simulink model "Control_test"  (R2014b)
settings: Solver=FixedStepDiscrete  StartTime=0.0  StopTime=Inf  FixedStep=0.001  RelTol=1e-3
PostLoadFcn:
  | , if any(exist('dsrtsu_mdlpostloadfcn', 'file') == [2, 3, 6]), try dsrtsu_mdlpostloadfcn('Execute', bdroot); catch fprintf('Error in PostLoadFcn (dsrtsu_mdlpostloadfcn) for model "%s":\n %s\n', bdroot, lasterr); end, end,
undefined symbols (not defined in the file or in its folder): dtLocal, slcm
libraries: rtican x163, simulink x14
(part 25 of 34)

== system Control_test/InputProcessing/RadarCanProcessing/Track39 ==
  Bus Creator : BusCreator  Inputs=12
  ESR_Track39 : rtican/RTICAN Receive (RX)   Reserved1=[]  Reserved2=[]  Reserved3=[]  Reserved4=[]  SfcnMessage=[]  Msg_Struct=[]  BoardTypeNo=[]  BoardNo=[]  ChannelNo=[]  Parameters=[]  DialogFcn=[]  UnitName=[]  Revision=[]  UnitValues=[]  DSProperties=struct('RTI',struct('Version',uint32(5),'BlockType',struct('isSLSource',uint8(1),'isSLSink',uint8(1),'isHWSource',uint8(0),'isHWSink',uint8(0),'isSetup',uint8(0),'isInline',uint8(1),'isNonInline',uint8(0),'isInterrupt',uint8(0),'isChannelwise',uint8(0)),'IOBoardType','RTICAN','UnitType','MESSAGE','Identifier','RX','DialogType','MSVC','BlockSet','RTICAN','SlaveProcessor','CAN'))  RTIBlockInterface=struct('OutputPortsWidth',int32([1 1 1 1 1 1 1 1 1 1 1 1]),'OutputPortsActive',[1 1 1 1 1 1 1 1 1 1 1 1],'OutputPortsName',{{'CAN_TX_TRACK_RANGE_RATE_39','CAN_TX_TRACK_MED_RANGE_MODE_39','CAN_TX_TRACK_RANGE_ACCEL_39','CAN_TX_TRACK_WIDTH_39','CAN_TX_TRACK_ROLLING_COUNT_39','CAN_TX_TRACK_BRIDGE_OBJECT_39','CAN_TX_TRACK_RANGE_39','CAN_TX_TRACK_ANGLE_39','CAN_TX_TRACK_STATUS_39','CAN_TX_TRACK_ONCOMING_39','CAN_TX_TRACK_GROUPING_CHANGED_39','CAN_TX_TRACK_LAT_RATE_39'}},'OutputPortsDataType',{{'SS_DOUBLE','SS_DOUBLE','SS_DOUBLE','SS_DOUBLE','SS_DOUBLE','SS_DOUBLE','SS_DOUBLE','SS_DOUBLE','SS_DOUBLE','SS_DOUBLE','SS_DOUBLE','SS_DOUBLE'}},'OutputPortsLabel',{{'CAN_TX_TRACK_RANGE_RATE_39','CAN_TX_TRACK_MED_RANGE_MODE_39','CAN_TX_TRACK_RANGE_ACCEL_39','CAN_TX_TRACK_WIDTH_39','CAN_TX_TRACK_ROLLING_COUNT_39','CAN_TX_TRACK_BRIDGE_OBJECT_39','CAN_TX_TRACK_RANGE_39','CAN_TX_TRACK_ANGLE_39','CAN_TX_TRACK_STATUS_39','CAN_TX_TRACK_ONCOMING_39','CAN_TX_TRACK_GROUPING_CHANGED_39','CAN_TX_TRACK_LAT_RATE_39'}},'OutputPortsLabelMode','ON','InputPortsWidth',int32(0),'InputPortsActive',0,'DialogFcn','rtican_message_interface_gui','BlockDisplay',{{'','center'}},'IconTransparency','on','ParameterTunableNames',{{}},'InitLevel',3,'BlockName',struct('Token',{{'ESR_Track39'}}),'SampleTime',{{0.01}},'TriggerPort',{{'none'}},'EnablePort',{{'none'}})  RTIBlockParameters=struct('BoardTypeNo',{{1,'OFF',[]}},'BoardNo',{{2,'ON',[1 16]}},'ChannelNo',{{2,'ON',[1 2]}},'Parameters',{{struct('DataFileSupport',struct('DataFileSelectedMaster',1,'DataFileSelectedLocal',0,'DataFileName','c:\users\mpc_car\documents\github\mpc-car\controller\dbcfiles\esr_dv3_64tgt.dbc|','DataFileDate',{{{['02-Nov-2012 20:32:52']},{['21-Mar-2013 13:39:53']},{['28-Sep-2011 17:08:52']}}},'SelectedFile',['<no file selected>'],'InterfaceFcn','rtican_dbc_file_parser'),'Options',struct('StatusSelected',0,'TimeSelected',0,'DeltaTimeSelected',0,'BytePortSelected',0,'MessageLengthSelected',0,'TriggerPort',struct('Selected',0,'TriggerType',0),'UserCoding',struct('Selected',0,'InterfaceFile','UserDecodingFile','FcnName','UserDecodeFcn','InportSelected',0,'InportWidth',1,'OutportSelected',0,'OutportWidth',1),'EnablePortSelected',0,'SignalOnPortnameSelected',1,'UseRXService',0),'Message',struct('MsgOnBlocknameSelected',1,'MsgName','ESR_Track39','MsgIdFormat',0,'MsgId',1318,'MsgLength',8,'NumSignals',12,'SampleTime',0.01,'Signal',struct('SgnName',{'CAN_TX_TRACK_RANGE_RATE_39','CAN_TX_TRACK_MED_RANGE_MODE_39','CAN_TX_TRACK_RANGE_ACCEL_39','CAN_TX_TRACK_WIDTH_39','CAN_TX_TRACK_ROLLING_COUNT_39','CAN_TX_TRACK_BRIDGE_OBJECT_39','CAN_TX_TRACK_RANGE_39','CAN_TX_TRACK_ANGLE_39','CAN_TX_TRACK_STATUS_39','CAN_TX_TRACK_ONCOMING_39','CAN_TX_TRACK_GROUPING_CHANGED_39','CAN_TX_TRACK_LAT_RATE_39'},'SgnStartBit',{0,14,16,26,30,31,32,43,53,56,57,58},'SgnLength',{14,2,10,4,1,1,11,10,3,1,1,6},'SgnType',{0,0,0,0,0,0,0,0,0,0,0,0},'ModeValue',{-1,-1,-1,-1,-1,-1,-1,-1,-1,-1,-1,-1},'DataType',{1,0,1,0,0,0,0,1,0,0,0,1},'ByteLayout',{2,2,2,2,2,2,2,2,2,2,2,2},'Factor',{0.01,1,0.05,0.5,1,1,0.1,0.1,1,1,1,0.25},'Offset',{0,0,0,0,0,0,0,0,0,0,0,0},'SgnComment',{{''},{''},{''},{''},{''},{''},{''},{''},{''},{''},{''},{''}},'SgnUnit',{'m/s','','m/s/s','m','','','m','deg','','','',''},'Min',{-81.92,0,-25.6,0,0,0,0,-51.2,0,0,0,-8},'Max',{81.91,3,25.55,7.5,1,0,204.7,51.1,7,0,0,7.75},'SLDataType',{'SS_DOUBLE','SS_DOUBLE','SS_DOUBLE','SS_DOUBLE','SS_DOUBLE','SS_DOUBLE','SS_DOUBLE','SS_DOUBLE','SS_DOUBLE','SS_DOUBLE','SS_DOUBLE','SS_DOUBLE'}),'MsgIdNumFormat',0,'MsgComment',{{''}}),'Version',1.2,'general',struct('isFromLib',0)),'OFF',[]}},'GroupId',{{struct('Group',{{'RTICAN'}},'No',4,'Behavior',{{'NAMECHANGE'}},'BlockType',{{'SINK'}},'NameChangeFlag',0),'OFF',[]}},'SFcnRTICANMessage',{{struct('MsgType','RX','SFcnPortType','Scalar','MsgName','ESR_Track39','MsgIdFormat','STD','MsgId',1318,'MsgLength',8,'NumSignals',12,'SampleTime',0.01,'Signal',struct('SgnName',{'CAN_TX_TRACK_RANGE_RATE_39','CAN_TX_TRACK_MED_RANGE_MODE_39','CAN_TX_TRACK_RANGE_ACCEL_39','CAN_TX_TRACK_WIDTH_39','CAN_TX_TRACK_ROLLING_COUNT_39','CAN_TX_TRACK_BRIDGE_OBJECT_39','CAN_TX_TRACK_RANGE_39','CAN_TX_TRACK_ANGLE_39','CAN_TX_TRACK_STATUS_39','CAN_TX_TRACK_ONCOMING_39','CAN_TX_TRACK_GROUPING_CHANGED_39','CAN_TX_TRACK_LAT_RATE_39'},'SgnStartBit',{0,14,16,26,30,31,32,43,53,56,57,58},'SgnLength',{14,2,10,4,1,1,11,10,3,1,1,6},'SgnType',{'standard','standard','standard','standard','standard','standard','standard','standard','standard','standard','standard','standard'},'ModeValue',{-1,-1,-1,-1,-1,-1,-1,-1,-1,-1,-1,-1},'DataType',{['signed int'],['unsigned int'],['signed int'],['unsigned int'],['unsigned int'],['unsigned int'],['unsigned int'],['signed int'],['unsigned int'],['unsigned int'],['unsigned int'],['signed int']},'ByteLayout',{['motorola back.'],['motorola back.'],['motorola back.'],['motorola back.'],['motorola back.'],['motorola back.'],['motorola back.'],['motorola back.'],['motorola back.'],['motorola back.'],['motorola back.'],['motorola back.']},'Factor',{0.01,1,0.05,0.5,1,1,0.1,0.1,1,1,1,0.25},'Offset',{0,0,0,0,0,0,0,0,0,0,0,0},'SLDataType',{'SS_DOUBLE','SS_DOUBLE','SS_DOUBLE','SS_DOUBLE','SS_DOUBLE','SS_DOUBLE','SS_DOUBLE','SS_DOUBLE','SS_DOUBLE','SS_DOUBLE','SS_DOUBLE','SS_DOUBLE'}),'StatusSelected','no','TimeSelected','no','DeltaTimeSelected','no','BytePortSelected','no','MessageLengthSelected','no','TriggerPort',struct('Selected','no','TriggerType',0),'UserCoding',struct('Selected','no','InterfaceFile','UserDecodingFile','FcnName','UserDecodeFcn','InportSelected','no','InportWidth',1,'OutportSelected','no','OutportWidth',1),'EnablePortSelected','no','UseRXService','no','BoardType','DS1','BoardNo',2,'ControllerNo',2),'OFF',[]}},'TLCFileName',{{'rtican_rx_message','OFF',[]}})  RTISFcnParameters=struct('SFcnRTICANMessage','struct','TLCFileName','char')  RTIBlockParaDefault=struct('BoardTypeNo',4302,'BoardNo',1,'ChannelNo',1,'Parameters',struct('DataFileSupport',struct('DataFileSelectedMaster',0,'DataFileSelectedLocal',0,'DataFileName','','DataFileDate','','SelectedFile',['<no file selected>']),'Options',struct('StatusSelected',1,'TimeSelected',1,'DeltaTimeSelected',1,'BytePortSelected',0,'MessageLengthSelected',0,'TriggerPort',struct('Selected',0,'TriggerType','rising'),'UserCoding',struct('Selected',0,'InterfaceFile','UserDecodingFile','FcnName','UserDecodeFcn','InportSelected',0,'InportWidth',1,'OutportSelected',0,'OutportWidth',1),'EnablePortSelected',0,'SignalOnPortnameSelected',1,'UseRXService',0),'Message',struct('MsgOnBlocknameSelected',0,'MsgName',['RX Message'],'MsgIdFormat',0,'MsgId',100,'MsgLength',8,'NumSignals',1,'SampleTime',-1,'Signal',struct('SgnName',['RX signal'],'SgnStartBit',0,'SgnLength',8,'SgnType',0,'ModeValue',-1,'DataType',0,'SLDataType','SS_DOUBLE','ByteLayout',0,'Factor',1,'Offset',0,'Min',0,'Max',255,'SgnComment',{{}},'SgnUnit',''),'MsgIdNumFormat',0,'MsgComment',{{''}}),'Version',1.2,'general',struct('isFromLib',1)),'GroupId',struct('Group',{{'RTICAN'}},'No',1,'Behavior',{{'NAMECHANGE'}},'BlockType',{{'SINK'}},'NameChangeFlag',0),'SFcnRTICANMessage',struct('MsgType','RX','MsgName',['RX Message'],'MsgIdFormat','STD','MsgId',100,'MsgLength',8,'NumSignals',1,'SampleTime',-1,'Signal',struct('SgnName',['RX signal'],'SgnStartBit',0,'SgnLength',8,'SgnType','standard','ModeValue',-1,'DataType',['unsigned int'],'ByteLayout',['little endian'],'SLDataType','SS_DOUBLE','Factor',1,'Offset',0),'StatusSelected','yes','TimeSelected','yes','DeltaTimeSelected','yes','BytePortSelected','no','MessageLengthSelected','no','EnablePortSelected','no','UserCoding',struct('Selected','no','InterfaceFile','UserDecodingFile','FcnName','UserDecodeFcn','InportSelected','no','InportWidth',1,'OutportSelected','no','OutportWidth',1),'TriggerPort',struct('Selected','no','TriggerType','rising'),'UseRXService','no','BoardType','DS4302','BoardNo',1,'ControllerNo',1,'SFcnPortType','Scalar'),'TLCFileName','rtican_rx_message')
      settings: AttributesFormatString=Group Id: RTICAN4\n
  Out1 : Outport
  wires:
  Bus Creator/1 -> Out1/1  "Track39"
  ESR_Track39/1 -> Bus Creator/1  "CAN_TX_TRACK_RANGE_RATE_39"
  ESR_Track39/2 -> Bus Creator/2  "CAN_TX_TRACK_MED_RANGE_MODE_39"
  ESR_Track39/3 -> Bus Creator/3  "CAN_TX_TRACK_RANGE_ACCEL_39"
  ESR_Track39/4 -> Bus Creator/4  "CAN_TX_TRACK_WIDTH_39"
  ESR_Track39/5 -> Bus Creator/5  "CAN_TX_TRACK_ROLLING_COUNT_39"
  ESR_Track39/6 -> Bus Creator/6  "CAN_TX_TRACK_BRIDGE_OBJECT_39"
  ESR_Track39/7 -> Bus Creator/7  "CAN_TX_TRACK_RANGE_39"
  ESR_Track39/8 -> Bus Creator/8  "CAN_TX_TRACK_ANGLE_39"
  ESR_Track39/9 -> Bus Creator/9  "CAN_TX_TRACK_STATUS_39"
  ESR_Track39/10 -> Bus Creator/10  "CAN_TX_TRACK_ONCOMING_39"
  ESR_Track39/11 -> Bus Creator/11  "CAN_TX_TRACK_GROUPING_CHANGED_39"
  ESR_Track39/12 -> Bus Creator/12  "CAN_TX_TRACK_LAT_RATE_39"

== system Control_test/InputProcessing/RadarCanProcessing/Track40 ==
  Bus Creator : BusCreator  Inputs=12
  ESR_Track40 : rtican/RTICAN Receive (RX)   Reserved1=[]  Reserved2=[]  Reserved3=[]  Reserved4=[]  SfcnMessage=[]  Msg_Struct=[]  BoardTypeNo=[]  BoardNo=[]  ChannelNo=[]  Parameters=[]  DialogFcn=[]  UnitName=[]  Revision=[]  UnitValues=[]  DSProperties=struct('RTI',struct('Version',uint32(5),'BlockType',struct('isSLSource',uint8(1),'isSLSink',uint8(1),'isHWSource',uint8(0),'isHWSink',uint8(0),'isSetup',uint8(0),'isInline',uint8(1),'isNonInline',uint8(0),'isInterrupt',uint8(0),'isChannelwise',uint8(0)),'IOBoardType','RTICAN','UnitType','MESSAGE','Identifier','RX','DialogType','MSVC','BlockSet','RTICAN','SlaveProcessor','CAN'))  RTIBlockInterface=struct('OutputPortsWidth',int32([1 1 1 1 1 1 1 1 1 1 1 1]),'OutputPortsActive',[1 1 1 1 1 1 1 1 1 1 1 1],'OutputPortsName',{{'CAN_TX_TRACK_RANGE_RATE_40','CAN_TX_TRACK_MED_RANGE_MODE_40','CAN_TX_TRACK_RANGE_ACCEL_40','CAN_TX_TRACK_WIDTH_40','CAN_TX_TRACK_ROLLING_COUNT_40','CAN_TX_TRACK_BRIDGE_OBJECT_40','CAN_TX_TRACK_RANGE_40','CAN_TX_TRACK_ANGLE_40','CAN_TX_TRACK_STATUS_40','CAN_TX_TRACK_ONCOMING_40','CAN_TX_TRACK_GROUPING_CHANGED_40','CAN_TX_TRACK_LAT_RATE_40'}},'OutputPortsDataType',{{'SS_DOUBLE','SS_DOUBLE','SS_DOUBLE','SS_DOUBLE','SS_DOUBLE','SS_DOUBLE','SS_DOUBLE','SS_DOUBLE','SS_DOUBLE','SS_DOUBLE','SS_DOUBLE','SS_DOUBLE'}},'OutputPortsLabel',{{'CAN_TX_TRACK_RANGE_RATE_40','CAN_TX_TRACK_MED_RANGE_MODE_40','CAN_TX_TRACK_RANGE_ACCEL_40','CAN_TX_TRACK_WIDTH_40','CAN_TX_TRACK_ROLLING_COUNT_40','CAN_TX_TRACK_BRIDGE_OBJECT_40','CAN_TX_TRACK_RANGE_40','CAN_TX_TRACK_ANGLE_40','CAN_TX_TRACK_STATUS_40','CAN_TX_TRACK_ONCOMING_40','CAN_TX_TRACK_GROUPING_CHANGED_40','CAN_TX_TRACK_LAT_RATE_40'}},'OutputPortsLabelMode','ON','InputPortsWidth',int32(0),'InputPortsActive',0,'DialogFcn','rtican_message_interface_gui','BlockDisplay',{{'','center'}},'IconTransparency','on','ParameterTunableNames',{{}},'InitLevel',3,'BlockName',struct('Token',{{'ESR_Track40'}}),'SampleTime',{{0.01}},'TriggerPort',{{'none'}},'EnablePort',{{'none'}})  RTIBlockParameters=struct('BoardTypeNo',{{1,'OFF',[]}},'BoardNo',{{2,'ON',[1 16]}},'ChannelNo',{{2,'ON',[1 2]}},'Parameters',{{struct('DataFileSupport',struct('DataFileSelectedMaster',1,'DataFileSelectedLocal',0,'DataFileName','c:\users\mpc_car\documents\github\mpc-car\controller\dbcfiles\esr_dv3_64tgt.dbc|','DataFileDate',{{{['02-Nov-2012 20:32:52']},{['21-Mar-2013 13:39:53']},{['28-Sep-2011 17:08:52']}}},'SelectedFile',['<no file selected>'],'InterfaceFcn','rtican_dbc_file_parser'),'Options',struct('StatusSelected',0,'TimeSelected',0,'DeltaTimeSelected',0,'BytePortSelected',0,'MessageLengthSelected',0,'TriggerPort',struct('Selected',0,'TriggerType',0),'UserCoding',struct('Selected',0,'InterfaceFile','UserDecodingFile','FcnName','UserDecodeFcn','InportSelected',0,'InportWidth',1,'OutportSelected',0,'OutportWidth',1),'EnablePortSelected',0,'SignalOnPortnameSelected',1,'UseRXService',0),'Message',struct('MsgOnBlocknameSelected',1,'MsgName','ESR_Track40','MsgIdFormat',0,'MsgId',1319,'MsgLength',8,'NumSignals',12,'SampleTime',0.01,'Signal',struct('SgnName',{'CAN_TX_TRACK_RANGE_RATE_40','CAN_TX_TRACK_MED_RANGE_MODE_40','CAN_TX_TRACK_RANGE_ACCEL_40','CAN_TX_TRACK_WIDTH_40','CAN_TX_TRACK_ROLLING_COUNT_40','CAN_TX_TRACK_BRIDGE_OBJECT_40','CAN_TX_TRACK_RANGE_40','CAN_TX_TRACK_ANGLE_40','CAN_TX_TRACK_STATUS_40','CAN_TX_TRACK_ONCOMING_40','CAN_TX_TRACK_GROUPING_CHANGED_40','CAN_TX_TRACK_LAT_RATE_40'},'SgnStartBit',{0,14,16,26,30,31,32,43,53,56,57,58},'SgnLength',{14,2,10,4,1,1,11,10,3,1,1,6},'SgnType',{0,0,0,0,0,0,0,0,0,0,0,0},'ModeValue',{-1,-1,-1,-1,-1,-1,-1,-1,-1,-1,-1,-1},'DataType',{1,0,1,0,0,0,0,1,0,0,0,1},'ByteLayout',{2,2,2,2,2,2,2,2,2,2,2,2},'Factor',{0.01,1,0.05,0.5,1,1,0.1,0.1,1,1,1,0.25},'Offset',{0,0,0,0,0,0,0,0,0,0,0,0},'SgnComment',{{''},{''},{''},{''},{''},{''},{''},{''},{''},{''},{''},{''}},'SgnUnit',{'m/s','','m/s/s','m','','','m','deg','','','',''},'Min',{-81.92,0,-25.6,0,0,0,0,-51.2,0,0,0,-8},'Max',{81.91,3,25.55,7.5,1,0,204.7,51.1,7,0,0,7.75},'SLDataType',{'SS_DOUBLE','SS_DOUBLE','SS_DOUBLE','SS_DOUBLE','SS_DOUBLE','SS_DOUBLE','SS_DOUBLE','SS_DOUBLE','SS_DOUBLE','SS_DOUBLE','SS_DOUBLE','SS_DOUBLE'}),'MsgIdNumFormat',0,'MsgComment',{{''}}),'Version',1.2,'general',struct('isFromLib',0)),'OFF',[]}},'GroupId',{{struct('Group',{{'RTICAN'}},'No',4,'Behavior',{{'NAMECHANGE'}},'BlockType',{{'SINK'}},'NameChangeFlag',0),'OFF',[]}},'SFcnRTICANMessage',{{struct('MsgType','RX','SFcnPortType','Scalar','MsgName','ESR_Track40','MsgIdFormat','STD','MsgId',1319,'MsgLength',8,'NumSignals',12,'SampleTime',0.01,'Signal',struct('SgnName',{'CAN_TX_TRACK_RANGE_RATE_40','CAN_TX_TRACK_MED_RANGE_MODE_40','CAN_TX_TRACK_RANGE_ACCEL_40','CAN_TX_TRACK_WIDTH_40','CAN_TX_TRACK_ROLLING_COUNT_40','CAN_TX_TRACK_BRIDGE_OBJECT_40','CAN_TX_TRACK_RANGE_40','CAN_TX_TRACK_ANGLE_40','CAN_TX_TRACK_STATUS_40','CAN_TX_TRACK_ONCOMING_40','CAN_TX_TRACK_GROUPING_CHANGED_40','CAN_TX_TRACK_LAT_RATE_40'},'SgnStartBit',{0,14,16,26,30,31,32,43,53,56,57,58},'SgnLength',{14,2,10,4,1,1,11,10,3,1,1,6},'SgnType',{'standard','standard','standard','standard','standard','standard','standard','standard','standard','standard','standard','standard'},'ModeValue',{-1,-1,-1,-1,-1,-1,-1,-1,-1,-1,-1,-1},'DataType',{['signed int'],['unsigned int'],['signed int'],['unsigned int'],['unsigned int'],['unsigned int'],['unsigned int'],['signed int'],['unsigned int'],['unsigned int'],['unsigned int'],['signed int']},'ByteLayout',{['motorola back.'],['motorola back.'],['motorola back.'],['motorola back.'],['motorola back.'],['motorola back.'],['motorola back.'],['motorola back.'],['motorola back.'],['motorola back.'],['motorola back.'],['motorola back.']},'Factor',{0.01,1,0.05,0.5,1,1,0.1,0.1,1,1,1,0.25},'Offset',{0,0,0,0,0,0,0,0,0,0,0,0},'SLDataType',{'SS_DOUBLE','SS_DOUBLE','SS_DOUBLE','SS_DOUBLE','SS_DOUBLE','SS_DOUBLE','SS_DOUBLE','SS_DOUBLE','SS_DOUBLE','SS_DOUBLE','SS_DOUBLE','SS_DOUBLE'}),'StatusSelected','no','TimeSelected','no','DeltaTimeSelected','no','BytePortSelected','no','MessageLengthSelected','no','TriggerPort',struct('Selected','no','TriggerType',0),'UserCoding',struct('Selected','no','InterfaceFile','UserDecodingFile','FcnName','UserDecodeFcn','InportSelected','no','InportWidth',1,'OutportSelected','no','OutportWidth',1),'EnablePortSelected','no','UseRXService','no','BoardType','DS1','BoardNo',2,'ControllerNo',2),'OFF',[]}},'TLCFileName',{{'rtican_rx_message','OFF',[]}})  RTISFcnParameters=struct('SFcnRTICANMessage','struct','TLCFileName','char')  RTIBlockParaDefault=struct('BoardTypeNo',4302,'BoardNo',1,'ChannelNo',1,'Parameters',struct('DataFileSupport',struct('DataFileSelectedMaster',0,'DataFileSelectedLocal',0,'DataFileName','','DataFileDate','','SelectedFile',['<no file selected>']),'Options',struct('StatusSelected',1,'TimeSelected',1,'DeltaTimeSelected',1,'BytePortSelected',0,'MessageLengthSelected',0,'TriggerPort',struct('Selected',0,'TriggerType','rising'),'UserCoding',struct('Selected',0,'InterfaceFile','UserDecodingFile','FcnName','UserDecodeFcn','InportSelected',0,'InportWidth',1,'OutportSelected',0,'OutportWidth',1),'EnablePortSelected',0,'SignalOnPortnameSelected',1,'UseRXService',0),'Message',struct('MsgOnBlocknameSelected',0,'MsgName',['RX Message'],'MsgIdFormat',0,'MsgId',100,'MsgLength',8,'NumSignals',1,'SampleTime',-1,'Signal',struct('SgnName',['RX signal'],'SgnStartBit',0,'SgnLength',8,'SgnType',0,'ModeValue',-1,'DataType',0,'SLDataType','SS_DOUBLE','ByteLayout',0,'Factor',1,'Offset',0,'Min',0,'Max',255,'SgnComment',{{}},'SgnUnit',''),'MsgIdNumFormat',0,'MsgComment',{{''}}),'Version',1.2,'general',struct('isFromLib',1)),'GroupId',struct('Group',{{'RTICAN'}},'No',1,'Behavior',{{'NAMECHANGE'}},'BlockType',{{'SINK'}},'NameChangeFlag',0),'SFcnRTICANMessage',struct('MsgType','RX','MsgName',['RX Message'],'MsgIdFormat','STD','MsgId',100,'MsgLength',8,'NumSignals',1,'SampleTime',-1,'Signal',struct('SgnName',['RX signal'],'SgnStartBit',0,'SgnLength',8,'SgnType','standard','ModeValue',-1,'DataType',['unsigned int'],'ByteLayout',['little endian'],'SLDataType','SS_DOUBLE','Factor',1,'Offset',0),'StatusSelected','yes','TimeSelected','yes','DeltaTimeSelected','yes','BytePortSelected','no','MessageLengthSelected','no','EnablePortSelected','no','UserCoding',struct('Selected','no','InterfaceFile','UserDecodingFile','FcnName','UserDecodeFcn','InportSelected','no','InportWidth',1,'OutportSelected','no','OutportWidth',1),'TriggerPort',struct('Selected','no','TriggerType','rising'),'UseRXService','no','BoardType','DS4302','BoardNo',1,'ControllerNo',1,'SFcnPortType','Scalar'),'TLCFileName','rtican_rx_message')
      settings: AttributesFormatString=Group Id: RTICAN4\n
  Out1 : Outport
  wires:
  Bus Creator/1 -> Out1/1  "Track40"
  ESR_Track40/1 -> Bus Creator/1  "CAN_TX_TRACK_RANGE_RATE_40"
  ESR_Track40/2 -> Bus Creator/2  "CAN_TX_TRACK_MED_RANGE_MODE_40"
  ESR_Track40/3 -> Bus Creator/3  "CAN_TX_TRACK_RANGE_ACCEL_40"
  ESR_Track40/4 -> Bus Creator/4  "CAN_TX_TRACK_WIDTH_40"
  ESR_Track40/5 -> Bus Creator/5  "CAN_TX_TRACK_ROLLING_COUNT_40"
  ESR_Track40/6 -> Bus Creator/6  "CAN_TX_TRACK_BRIDGE_OBJECT_40"
  ESR_Track40/7 -> Bus Creator/7  "CAN_TX_TRACK_RANGE_40"
  ESR_Track40/8 -> Bus Creator/8  "CAN_TX_TRACK_ANGLE_40"
  ESR_Track40/9 -> Bus Creator/9  "CAN_TX_TRACK_STATUS_40"
  ESR_Track40/10 -> Bus Creator/10  "CAN_TX_TRACK_ONCOMING_40"
  ESR_Track40/11 -> Bus Creator/11  "CAN_TX_TRACK_GROUPING_CHANGED_40"
  ESR_Track40/12 -> Bus Creator/12  "CAN_TX_TRACK_LAT_RATE_40"

== system Control_test/InputProcessing/RadarCanProcessing/Track41 ==
  Bus Creator : BusCreator  Inputs=12
  ESR_Track41 : rtican/RTICAN Receive (RX)   Reserved1=[]  Reserved2=[]  Reserved3=[]  Reserved4=[]  SfcnMessage=[]  Msg_Struct=[]  BoardTypeNo=[]  BoardNo=[]  ChannelNo=[]  Parameters=[]  DialogFcn=[]  UnitName=[]  Revision=[]  UnitValues=[]  DSProperties=struct('RTI',struct('Version',uint32(5),'BlockType',struct('isSLSource',uint8(1),'isSLSink',uint8(1),'isHWSource',uint8(0),'isHWSink',uint8(0),'isSetup',uint8(0),'isInline',uint8(1),'isNonInline',uint8(0),'isInterrupt',uint8(0),'isChannelwise',uint8(0)),'IOBoardType','RTICAN','UnitType','MESSAGE','Identifier','RX','DialogType','MSVC','BlockSet','RTICAN','SlaveProcessor','CAN'))  RTIBlockInterface=struct('OutputPortsWidth',int32([1 1 1 1 1 1 1 1 1 1 1 1]),'OutputPortsActive',[1 1 1 1 1 1 1 1 1 1 1 1],'OutputPortsName',{{'CAN_TX_TRACK_RANGE_RATE_41','CAN_TX_TRACK_MED_RANGE_MODE_41','CAN_TX_TRACK_RANGE_ACCEL_41','CAN_TX_TRACK_WIDTH_41','CAN_TX_TRACK_ROLLING_COUNT_41','CAN_TX_TRACK_BRIDGE_OBJECT_41','CAN_TX_TRACK_RANGE_41','CAN_TX_TRACK_ANGLE_41','CAN_TX_TRACK_STATUS_41','CAN_TX_TRACK_ONCOMING_41','CAN_TX_TRACK_GROUPING_CHANGED_41','CAN_TX_TRACK_LAT_RATE_41'}},'OutputPortsDataType',{{'SS_DOUBLE','SS_DOUBLE','SS_DOUBLE','SS_DOUBLE','SS_DOUBLE','SS_DOUBLE','SS_DOUBLE','SS_DOUBLE','SS_DOUBLE','SS_DOUBLE','SS_DOUBLE','SS_DOUBLE'}},'OutputPortsLabel',{{'CAN_TX_TRACK_RANGE_RATE_41','CAN_TX_TRACK_MED_RANGE_MODE_41','CAN_TX_TRACK_RANGE_ACCEL_41','CAN_TX_TRACK_WIDTH_41','CAN_TX_TRACK_ROLLING_COUNT_41','CAN_TX_TRACK_BRIDGE_OBJECT_41','CAN_TX_TRACK_RANGE_41','CAN_TX_TRACK_ANGLE_41','CAN_TX_TRACK_STATUS_41','CAN_TX_TRACK_ONCOMING_41','CAN_TX_TRACK_GROUPING_CHANGED_41','CAN_TX_TRACK_LAT_RATE_41'}},'OutputPortsLabelMode','ON','InputPortsWidth',int32(0),'InputPortsActive',0,'DialogFcn','rtican_message_interface_gui','BlockDisplay',{{'','center'}},'IconTransparency','on','ParameterTunableNames',{{}},'InitLevel',3,'BlockName',struct('Token',{{'ESR_Track41'}}),'SampleTime',{{0.01}},'TriggerPort',{{'none'}},'EnablePort',{{'none'}})  RTIBlockParameters=struct('BoardTypeNo',{{1,'OFF',[]}},'BoardNo',{{2,'ON',[1 16]}},'ChannelNo',{{2,'ON',[1 2]}},'Parameters',{{struct('DataFileSupport',struct('DataFileSelectedMaster',1,'DataFileSelectedLocal',0,'DataFileName','c:\users\mpc_car\documents\github\mpc-car\controller\dbcfiles\esr_dv3_64tgt.dbc|','DataFileDate',{{{['02-Nov-2012 20:32:52']},{['21-Mar-2013 13:39:53']},{['28-Sep-2011 17:08:52']}}},'SelectedFile',['<no file selected>'],'InterfaceFcn','rtican_dbc_file_parser'),'Options',struct('StatusSelected',0,'TimeSelected',0,'DeltaTimeSelected',0,'BytePortSelected',0,'MessageLengthSelected',0,'TriggerPort',struct('Selected',0,'TriggerType',0),'UserCoding',struct('Selected',0,'InterfaceFile','UserDecodingFile','FcnName','UserDecodeFcn','InportSelected',0,'InportWidth',1,'OutportSelected',0,'OutportWidth',1),'EnablePortSelected',0,'SignalOnPortnameSelected',1,'UseRXService',0),'Message',struct('MsgOnBlocknameSelected',1,'MsgName','ESR_Track41','MsgIdFormat',0,'MsgId',1320,'MsgLength',8,'NumSignals',12,'SampleTime',0.01,'Signal',struct('SgnName',{'CAN_TX_TRACK_RANGE_RATE_41','CAN_TX_TRACK_MED_RANGE_MODE_41','CAN_TX_TRACK_RANGE_ACCEL_41','CAN_TX_TRACK_WIDTH_41','CAN_TX_TRACK_ROLLING_COUNT_41','CAN_TX_TRACK_BRIDGE_OBJECT_41','CAN_TX_TRACK_RANGE_41','CAN_TX_TRACK_ANGLE_41','CAN_TX_TRACK_STATUS_41','CAN_TX_TRACK_ONCOMING_41','CAN_TX_TRACK_GROUPING_CHANGED_41','CAN_TX_TRACK_LAT_RATE_41'},'SgnStartBit',{0,14,16,26,30,31,32,43,53,56,57,58},'SgnLength',{14,2,10,4,1,1,11,10,3,1,1,6},'SgnType',{0,0,0,0,0,0,0,0,0,0,0,0},'ModeValue',{-1,-1,-1,-1,-1,-1,-1,-1,-1,-1,-1,-1},'DataType',{1,0,1,0,0,0,0,1,0,0,0,1},'ByteLayout',{2,2,2,2,2,2,2,2,2,2,2,2},'Factor',{0.01,1,0.05,0.5,1,1,0.1,0.1,1,1,1,0.25},'Offset',{0,0,0,0,0,0,0,0,0,0,0,0},'SgnComment',{{''},{''},{''},{''},{''},{''},{''},{''},{''},{''},{''},{''}},'SgnUnit',{'m/s','','m/s/s','m','','','m','deg','','','',''},'Min',{-81.92,0,-25.6,0,0,0,0,-51.2,0,0,0,-8},'Max',{81.91,3,25.55,7.5,1,0,204.7,51.1,7,0,0,7.75},'SLDataType',{'SS_DOUBLE','SS_DOUBLE','SS_DOUBLE','SS_DOUBLE','SS_DOUBLE','SS_DOUBLE','SS_DOUBLE','SS_DOUBLE','SS_DOUBLE','SS_DOUBLE','SS_DOUBLE','SS_DOUBLE'}),'MsgIdNumFormat',0,'MsgComment',{{''}}),'Version',1.2,'general',struct('isFromLib',0)),'OFF',[]}},'GroupId',{{struct('Group',{{'RTICAN'}},'No',4,'Behavior',{{'NAMECHANGE'}},'BlockType',{{'SINK'}},'NameChangeFlag',0),'OFF',[]}},'SFcnRTICANMessage',{{struct('MsgType','RX','SFcnPortType','Scalar','MsgName','ESR_Track41','MsgIdFormat','STD','MsgId',1320,'MsgLength',8,'NumSignals',12,'SampleTime',0.01,'Signal',struct('SgnName',{'CAN_TX_TRACK_RANGE_RATE_41','CAN_TX_TRACK_MED_RANGE_MODE_41','CAN_TX_TRACK_RANGE_ACCEL_41','CAN_TX_TRACK_WIDTH_41','CAN_TX_TRACK_ROLLING_COUNT_41','CAN_TX_TRACK_BRIDGE_OBJECT_41','CAN_TX_TRACK_RANGE_41','CAN_TX_TRACK_ANGLE_41','CAN_TX_TRACK_STATUS_41','CAN_TX_TRACK_ONCOMING_41','CAN_TX_TRACK_GROUPING_CHANGED_41','CAN_TX_TRACK_LAT_RATE_41'},'SgnStartBit',{0,14,16,26,30,31,32,43,53,56,57,58},'SgnLength',{14,2,10,4,1,1,11,10,3,1,1,6},'SgnType',{'standard','standard','standard','standard','standard','standard','standard','standard','standard','standard','standard','standard'},'ModeValue',{-1,-1,-1,-1,-1,-1,-1,-1,-1,-1,-1,-1},'DataType',{['signed int'],['unsigned int'],['signed int'],['unsigned int'],['unsigned int'],['unsigned int'],['unsigned int'],['signed int'],['unsigned int'],['unsigned int'],['unsigned int'],['signed int']},'ByteLayout',{['motorola back.'],['motorola back.'],['motorola back.'],['motorola back.'],['motorola back.'],['motorola back.'],['motorola back.'],['motorola back.'],['motorola back.'],['motorola back.'],['motorola back.'],['motorola back.']},'Factor',{0.01,1,0.05,0.5,1,1,0.1,0.1,1,1,1,0.25},'Offset',{0,0,0,0,0,0,0,0,0,0,0,0},'SLDataType',{'SS_DOUBLE','SS_DOUBLE','SS_DOUBLE','SS_DOUBLE','SS_DOUBLE','SS_DOUBLE','SS_DOUBLE','SS_DOUBLE','SS_DOUBLE','SS_DOUBLE','SS_DOUBLE','SS_DOUBLE'}),'StatusSelected','no','TimeSelected','no','DeltaTimeSelected','no','BytePortSelected','no','MessageLengthSelected','no','TriggerPort',struct('Selected','no','TriggerType',0),'UserCoding',struct('Selected','no','InterfaceFile','UserDecodingFile','FcnName','UserDecodeFcn','InportSelected','no','InportWidth',1,'OutportSelected','no','OutportWidth',1),'EnablePortSelected','no','UseRXService','no','BoardType','DS1','BoardNo',2,'ControllerNo',2),'OFF',[]}},'TLCFileName',{{'rtican_rx_message','OFF',[]}})  RTISFcnParameters=struct('SFcnRTICANMessage','struct','TLCFileName','char')  RTIBlockParaDefault=struct('BoardTypeNo',4302,'BoardNo',1,'ChannelNo',1,'Parameters',struct('DataFileSupport',struct('DataFileSelectedMaster',0,'DataFileSelectedLocal',0,'DataFileName','','DataFileDate','','SelectedFile',['<no file selected>']),'Options',struct('StatusSelected',1,'TimeSelected',1,'DeltaTimeSelected',1,'BytePortSelected',0,'MessageLengthSelected',0,'TriggerPort',struct('Selected',0,'TriggerType','rising'),'UserCoding',struct('Selected',0,'InterfaceFile','UserDecodingFile','FcnName','UserDecodeFcn','InportSelected',0,'InportWidth',1,'OutportSelected',0,'OutportWidth',1),'EnablePortSelected',0,'SignalOnPortnameSelected',1,'UseRXService',0),'Message',struct('MsgOnBlocknameSelected',0,'MsgName',['RX Message'],'MsgIdFormat',0,'MsgId',100,'MsgLength',8,'NumSignals',1,'SampleTime',-1,'Signal',struct('SgnName',['RX signal'],'SgnStartBit',0,'SgnLength',8,'SgnType',0,'ModeValue',-1,'DataType',0,'SLDataType','SS_DOUBLE','ByteLayout',0,'Factor',1,'Offset',0,'Min',0,'Max',255,'SgnComment',{{}},'SgnUnit',''),'MsgIdNumFormat',0,'MsgComment',{{''}}),'Version',1.2,'general',struct('isFromLib',1)),'GroupId',struct('Group',{{'RTICAN'}},'No',1,'Behavior',{{'NAMECHANGE'}},'BlockType',{{'SINK'}},'NameChangeFlag',0),'SFcnRTICANMessage',struct('MsgType','RX','MsgName',['RX Message'],'MsgIdFormat','STD','MsgId',100,'MsgLength',8,'NumSignals',1,'SampleTime',-1,'Signal',struct('SgnName',['RX signal'],'SgnStartBit',0,'SgnLength',8,'SgnType','standard','ModeValue',-1,'DataType',['unsigned int'],'ByteLayout',['little endian'],'SLDataType','SS_DOUBLE','Factor',1,'Offset',0),'StatusSelected','yes','TimeSelected','yes','DeltaTimeSelected','yes','BytePortSelected','no','MessageLengthSelected','no','EnablePortSelected','no','UserCoding',struct('Selected','no','InterfaceFile','UserDecodingFile','FcnName','UserDecodeFcn','InportSelected','no','InportWidth',1,'OutportSelected','no','OutportWidth',1),'TriggerPort',struct('Selected','no','TriggerType','rising'),'UseRXService','no','BoardType','DS4302','BoardNo',1,'ControllerNo',1,'SFcnPortType','Scalar'),'TLCFileName','rtican_rx_message')
      settings: AttributesFormatString=Group Id: RTICAN4\n
  Out1 : Outport
  wires:
  Bus Creator/1 -> Out1/1  "Track41"
  ESR_Track41/1 -> Bus Creator/1  "CAN_TX_TRACK_RANGE_RATE_41"
  ESR_Track41/2 -> Bus Creator/2  "CAN_TX_TRACK_MED_RANGE_MODE_41"
  ESR_Track41/3 -> Bus Creator/3  "CAN_TX_TRACK_RANGE_ACCEL_41"
  ESR_Track41/4 -> Bus Creator/4  "CAN_TX_TRACK_WIDTH_41"
  ESR_Track41/5 -> Bus Creator/5  "CAN_TX_TRACK_ROLLING_COUNT_41"
  ESR_Track41/6 -> Bus Creator/6  "CAN_TX_TRACK_BRIDGE_OBJECT_41"
  ESR_Track41/7 -> Bus Creator/7  "CAN_TX_TRACK_RANGE_41"
  ESR_Track41/8 -> Bus Creator/8  "CAN_TX_TRACK_ANGLE_41"
  ESR_Track41/9 -> Bus Creator/9  "CAN_TX_TRACK_STATUS_41"
  ESR_Track41/10 -> Bus Creator/10  "CAN_TX_TRACK_ONCOMING_41"
  ESR_Track41/11 -> Bus Creator/11  "CAN_TX_TRACK_GROUPING_CHANGED_41"
  ESR_Track41/12 -> Bus Creator/12  "CAN_TX_TRACK_LAT_RATE_41"

== system Control_test/InputProcessing/RadarCanProcessing/Track42 ==
  Bus Creator : BusCreator  Inputs=12
  ESR_Track42 : rtican/RTICAN Receive (RX)   Reserved1=[]  Reserved2=[]  Reserved3=[]  Reserved4=[]  SfcnMessage=[]  Msg_Struct=[]  BoardTypeNo=[]  BoardNo=[]  ChannelNo=[]  Parameters=[]  DialogFcn=[]  UnitName=[]  Revision=[]  UnitValues=[]  DSProperties=struct('RTI',struct('Version',uint32(5),'BlockType',struct('isSLSource',uint8(1),'isSLSink',uint8(1),'isHWSource',uint8(0),'isHWSink',uint8(0),'isSetup',uint8(0),'isInline',uint8(1),'isNonInline',uint8(0),'isInterrupt',uint8(0),'isChannelwise',uint8(0)),'IOBoardType','RTICAN','UnitType','MESSAGE','Identifier','RX','DialogType','MSVC','BlockSet','RTICAN','SlaveProcessor','CAN'))  RTIBlockInterface=struct('OutputPortsWidth',int32([1 1 1 1 1 1 1 1 1 1 1 1]),'OutputPortsActive',[1 1 1 1 1 1 1 1 1 1 1 1],'OutputPortsName',{{'CAN_TX_TRACK_RANGE_RATE_42','CAN_TX_TRACK_MED_RANGE_MODE_42','CAN_TX_TRACK_RANGE_ACCEL_42','CAN_TX_TRACK_WIDTH_42','CAN_TX_TRACK_ROLLING_COUNT_42','CAN_TX_TRACK_BRIDGE_OBJECT_42','CAN_TX_TRACK_RANGE_42','CAN_TX_TRACK_ANGLE_42','CAN_TX_TRACK_STATUS_42','CAN_TX_TRACK_ONCOMING_42','CAN_TX_TRACK_GROUPING_CHANGED_42','CAN_TX_TRACK_LAT_RATE_42'}},'OutputPortsDataType',{{'SS_DOUBLE','SS_DOUBLE','SS_DOUBLE','SS_DOUBLE','SS_DOUBLE','SS_DOUBLE','SS_DOUBLE','SS_DOUBLE','SS_DOUBLE','SS_DOUBLE','SS_DOUBLE','SS_DOUBLE'}},'OutputPortsLabel',{{'CAN_TX_TRACK_RANGE_RATE_42','CAN_TX_TRACK_MED_RANGE_MODE_42','CAN_TX_TRACK_RANGE_ACCEL_42','CAN_TX_TRACK_WIDTH_42','CAN_TX_TRACK_ROLLING_COUNT_42','CAN_TX_TRACK_BRIDGE_OBJECT_42','CAN_TX_TRACK_RANGE_42','CAN_TX_TRACK_ANGLE_42','CAN_TX_TRACK_STATUS_42','CAN_TX_TRACK_ONCOMING_42','CAN_TX_TRACK_GROUPING_CHANGED_42','CAN_TX_TRACK_LAT_RATE_42'}},'OutputPortsLabelMode','ON','InputPortsWidth',int32(0),'InputPortsActive',0,'DialogFcn','rtican_message_interface_gui','BlockDisplay',{{'','center'}},'IconTransparency','on','ParameterTunableNames',{{}},'InitLevel',3,'BlockName',struct('Token',{{'ESR_Track42'}}),'SampleTime',{{0.01}},'TriggerPort',{{'none'}},'EnablePort',{{'none'}})  RTIBlockParameters=struct('BoardTypeNo',{{1,'OFF',[]}},'BoardNo',{{2,'ON',[1 16]}},'ChannelNo',{{2,'ON',[1 2]}},'Parameters',{{struct('DataFileSupport',struct('DataFileSelectedMaster',1,'DataFileSelectedLocal',0,'DataFileName','c:\users\mpc_car\documents\github\mpc-car\controller\dbcfiles\esr_dv3_64tgt.dbc|','DataFileDate',{{{['02-Nov-2012 20:32:52']},{['21-Mar-2013 13:39:53']},{['28-Sep-2011 17:08:52']}}},'SelectedFile',['<no file selected>'],'InterfaceFcn','rtican_dbc_file_parser'),'Options',struct('StatusSelected',0,'TimeSelected',0,'DeltaTimeSelected',0,'BytePortSelected',0,'MessageLengthSelected',0,'TriggerPort',struct('Selected',0,'TriggerType',0),'UserCoding',struct('Selected',0,'InterfaceFile','UserDecodingFile','FcnName','UserDecodeFcn','InportSelected',0,'InportWidth',1,'OutportSelected',0,'OutportWidth',1),'EnablePortSelected',0,'SignalOnPortnameSelected',1,'UseRXService',0),'Message',struct('MsgOnBlocknameSelected',1,'MsgName','ESR_Track42','MsgIdFormat',0,'MsgId',1321,'MsgLength',8,'NumSignals',12,'SampleTime',0.01,'Signal',struct('SgnName',{'CAN_TX_TRACK_RANGE_RATE_42','CAN_TX_TRACK_MED_RANGE_MODE_42','CAN_TX_TRACK_RANGE_ACCEL_42','CAN_TX_TRACK_WIDTH_42','CAN_TX_TRACK_ROLLING_COUNT_42','CAN_TX_TRACK_BRIDGE_OBJECT_42','CAN_TX_TRACK_RANGE_42','CAN_TX_TRACK_ANGLE_42','CAN_TX_TRACK_STATUS_42','CAN_TX_TRACK_ONCOMING_42','CAN_TX_TRACK_GROUPING_CHANGED_42','CAN_TX_TRACK_LAT_RATE_42'},'SgnStartBit',{0,14,16,26,30,31,32,43,53,56,57,58},'SgnLength',{14,2,10,4,1,1,11,10,3,1,1,6},'SgnType',{0,0,0,0,0,0,0,0,0,0,0,0},'ModeValue',{-1,-1,-1,-1,-1,-1,-1,-1,-1,-1,-1,-1},'DataType',{1,0,1,0,0,0,0,1,0,0,0,1},'ByteLayout',{2,2,2,2,2,2,2,2,2,2,2,2},'Factor',{0.01,1,0.05,0.5,1,1,0.1,0.1,1,1,1,0.25},'Offset',{0,0,0,0,0,0,0,0,0,0,0,0},'SgnComment',{{''},{''},{''},{''},{''},{''},{''},{''},{''},{''},{''},{''}},'SgnUnit',{'m/s','','m/s/s','m','','','m','deg','','','',''},'Min',{-81.92,0,-25.6,0,0,0,0,-51.2,0,0,0,-8},'Max',{81.91,3,25.55,7.5,1,0,204.7,51.1,7,0,0,7.75},'SLDataType',{'SS_DOUBLE','SS_DOUBLE','SS_DOUBLE','SS_DOUBLE','SS_DOUBLE','SS_DOUBLE','SS_DOUBLE','SS_DOUBLE','SS_DOUBLE','SS_DOUBLE','SS_DOUBLE','SS_DOUBLE'}),'MsgIdNumFormat',0,'MsgComment',{{''}}),'Version',1.2,'general',struct('isFromLib',0)),'OFF',[]}},'GroupId',{{struct('Group',{{'RTICAN'}},'No',4,'Behavior',{{'NAMECHANGE'}},'BlockType',{{'SINK'}},'NameChangeFlag',0),'OFF',[]}},'SFcnRTICANMessage',{{struct('MsgType','RX','SFcnPortType','Scalar','MsgName','ESR_Track42','MsgIdFormat','STD','MsgId',1321,'MsgLength',8,'NumSignals',12,'SampleTime',0.01,'Signal',struct('SgnName',{'CAN_TX_TRACK_RANGE_RATE_42','CAN_TX_TRACK_MED_RANGE_MODE_42','CAN_TX_TRACK_RANGE_ACCEL_42','CAN_TX_TRACK_WIDTH_42','CAN_TX_TRACK_ROLLING_COUNT_42','CAN_TX_TRACK_BRIDGE_OBJECT_42','CAN_TX_TRACK_RANGE_42','CAN_TX_TRACK_ANGLE_42','CAN_TX_TRACK_STATUS_42','CAN_TX_TRACK_ONCOMING_42','CAN_TX_TRACK_GROUPING_CHANGED_42','CAN_TX_TRACK_LAT_RATE_42'},'SgnStartBit',{0,14,16,26,30,31,32,43,53,56,57,58},'SgnLength',{14,2,10,4,1,1,11,10,3,1,1,6},'SgnType',{'standard','standard','standard','standard','standard','standard','standard','standard','standard','standard','standard','standard'},'ModeValue',{-1,-1,-1,-1,-1,-1,-1,-1,-1,-1,-1,-1},'DataType',{['signed int'],['unsigned int'],['signed int'],['unsigned int'],['unsigned int'],['unsigned int'],['unsigned int'],['signed int'],['unsigned int'],['unsigned int'],['unsigned int'],['signed int']},'ByteLayout',{['motorola back.'],['motorola back.'],['motorola back.'],['motorola back.'],['motorola back.'],['motorola back.'],['motorola back.'],['motorola back.'],['motorola back.'],['motorola back.'],['motorola back.'],['motorola back.']},'Factor',{0.01,1,0.05,0.5,1,1,0.1,0.1,1,1,1,0.25},'Offset',{0,0,0,0,0,0,0,0,0,0,0,0},'SLDataType',{'SS_DOUBLE','SS_DOUBLE','SS_DOUBLE','SS_DOUBLE','SS_DOUBLE','SS_DOUBLE','SS_DOUBLE','SS_DOUBLE','SS_DOUBLE','SS_DOUBLE','SS_DOUBLE','SS_DOUBLE'}),'StatusSelected','no','TimeSelected','no','DeltaTimeSelected','no','BytePortSelected','no','MessageLengthSelected','no','TriggerPort',struct('Selected','no','TriggerType',0),'UserCoding',struct('Selected','no','InterfaceFile','UserDecodingFile','FcnName','UserDecodeFcn','InportSelected','no','InportWidth',1,'OutportSelected','no','OutportWidth',1),'EnablePortSelected','no','UseRXService','no','BoardType','DS1','BoardNo',2,'ControllerNo',2),'OFF',[]}},'TLCFileName',{{'rtican_rx_message','OFF',[]}})  RTISFcnParameters=struct('SFcnRTICANMessage','struct','TLCFileName','char')  RTIBlockParaDefault=struct('BoardTypeNo',4302,'BoardNo',1,'ChannelNo',1,'Parameters',struct('DataFileSupport',struct('DataFileSelectedMaster',0,'DataFileSelectedLocal',0,'DataFileName','','DataFileDate','','SelectedFile',['<no file selected>']),'Options',struct('StatusSelected',1,'TimeSelected',1,'DeltaTimeSelected',1,'BytePortSelected',0,'MessageLengthSelected',0,'TriggerPort',struct('Selected',0,'TriggerType','rising'),'UserCoding',struct('Selected',0,'InterfaceFile','UserDecodingFile','FcnName','UserDecodeFcn','InportSelected',0,'InportWidth',1,'OutportSelected',0,'OutportWidth',1),'EnablePortSelected',0,'SignalOnPortnameSelected',1,'UseRXService',0),'Message',struct('MsgOnBlocknameSelected',0,'MsgName',['RX Message'],'MsgIdFormat',0,'MsgId',100,'MsgLength',8,'NumSignals',1,'SampleTime',-1,'Signal',struct('SgnName',['RX signal'],'SgnStartBit',0,'SgnLength',8,'SgnType',0,'ModeValue',-1,'DataType',0,'SLDataType','SS_DOUBLE','ByteLayout',0,'Factor',1,'Offset',0,'Min',0,'Max',255,'SgnComment',{{}},'SgnUnit',''),'MsgIdNumFormat',0,'MsgComment',{{''}}),'Version',1.2,'general',struct('isFromLib',1)),'GroupId',struct('Group',{{'RTICAN'}},'No',1,'Behavior',{{'NAMECHANGE'}},'BlockType',{{'SINK'}},'NameChangeFlag',0),'SFcnRTICANMessage',struct('MsgType','RX','MsgName',['RX Message'],'MsgIdFormat','STD','MsgId',100,'MsgLength',8,'NumSignals',1,'SampleTime',-1,'Signal',struct('SgnName',['RX signal'],'SgnStartBit',0,'SgnLength',8,'SgnType','standard','ModeValue',-1,'DataType',['unsigned int'],'ByteLayout',['little endian'],'SLDataType','SS_DOUBLE','Factor',1,'Offset',0),'StatusSelected','yes','TimeSelected','yes','DeltaTimeSelected','yes','BytePortSelected','no','MessageLengthSelected','no','EnablePortSelected','no','UserCoding',struct('Selected','no','InterfaceFile','UserDecodingFile','FcnName','UserDecodeFcn','InportSelected','no','InportWidth',1,'OutportSelected','no','OutportWidth',1),'TriggerPort',struct('Selected','no','TriggerType','rising'),'UseRXService','no','BoardType','DS4302','BoardNo',1,'ControllerNo',1,'SFcnPortType','Scalar'),'TLCFileName','rtican_rx_message')
      settings: AttributesFormatString=Group Id: RTICAN4\n
  Out1 : Outport
  wires:
  Bus Creator/1 -> Out1/1  "Track42"
  ESR_Track42/1 -> Bus Creator/1  "CAN_TX_TRACK_RANGE_RATE_42"
  ESR_Track42/2 -> Bus Creator/2  "CAN_TX_TRACK_MED_RANGE_MODE_42"
  ESR_Track42/3 -> Bus Creator/3  "CAN_TX_TRACK_RANGE_ACCEL_42"
  ESR_Track42/4 -> Bus Creator/4  "CAN_TX_TRACK_WIDTH_42"
  ESR_Track42/5 -> Bus Creator/5  "CAN_TX_TRACK_ROLLING_COUNT_42"
  ESR_Track42/6 -> Bus Creator/6  "CAN_TX_TRACK_BRIDGE_OBJECT_42"
  ESR_Track42/7 -> Bus Creator/7  "CAN_TX_TRACK_RANGE_42"
  ESR_Track42/8 -> Bus Creator/8  "CAN_TX_TRACK_ANGLE_42"
  ESR_Track42/9 -> Bus Creator/9  "CAN_TX_TRACK_STATUS_42"
  ESR_Track42/10 -> Bus Creator/10  "CAN_TX_TRACK_ONCOMING_42"
  ESR_Track42/11 -> Bus Creator/11  "CAN_TX_TRACK_GROUPING_CHANGED_42"
  ESR_Track42/12 -> Bus Creator/12  "CAN_TX_TRACK_LAT_RATE_42"

== system Control_test/InputProcessing/RadarCanProcessing/Track43 ==
  Bus Creator : BusCreator  Inputs=12
  ESR_Track43 : rtican/RTICAN Receive (RX)   Reserved1=[]  Reserved2=[]  Reserved3=[]  Reserved4=[]  SfcnMessage=[]  Msg_Struct=[]  BoardTypeNo=[]  BoardNo=[]  ChannelNo=[]  Parameters=[]  DialogFcn=[]  UnitName=[]  Revision=[]  UnitValues=[]  DSProperties=struct('RTI',struct('Version',uint32(5),'BlockType',struct('isSLSource',uint8(1),'isSLSink',uint8(1),'isHWSource',uint8(0),'isHWSink',uint8(0),'isSetup',uint8(0),'isInline',uint8(1),'isNonInline',uint8(0),'isInterrupt',uint8(0),'isChannelwise',uint8(0)),'IOBoardType','RTICAN','UnitType','MESSAGE','Identifier','RX','DialogType','MSVC','BlockSet','RTICAN','SlaveProcessor','CAN'))  RTIBlockInterface=struct('OutputPortsWidth',int32([1 1 1 1 1 1 1 1 1 1 1 1]),'OutputPortsActive',[1 1 1 1 1 1 1 1 1 1 1 1],'OutputPortsName',{{'CAN_TX_TRACK_RANGE_RATE_43','CAN_TX_TRACK_MED_RANGE_MODE_43','CAN_TX_TRACK_RANGE_ACCEL_43','CAN_TX_TRACK_WIDTH_43','CAN_TX_TRACK_ROLLING_COUNT_43','CAN_TX_TRACK_BRIDGE_OBJECT_43','CAN_TX_TRACK_RANGE_43','CAN_TX_TRACK_ANGLE_43','CAN_TX_TRACK_STATUS_43','CAN_TX_TRACK_ONCOMING_43','CAN_TX_TRACK_GROUPING_CHANGED_43','CAN_TX_TRACK_LAT_RATE_43'}},'OutputPortsDataType',{{'SS_DOUBLE','SS_DOUBLE','SS_DOUBLE','SS_DOUBLE','SS_DOUBLE','SS_DOUBLE','SS_DOUBLE','SS_DOUBLE','SS_DOUBLE','SS_DOUBLE','SS_DOUBLE','SS_DOUBLE'}},'OutputPortsLabel',{{'CAN_TX_TRACK_RANGE_RATE_43','CAN_TX_TRACK_MED_RANGE_MODE_43','CAN_TX_TRACK_RANGE_ACCEL_43','CAN_TX_TRACK_WIDTH_43','CAN_TX_TRACK_ROLLING_COUNT_43','CAN_TX_TRACK_BRIDGE_OBJECT_43','CAN_TX_TRACK_RANGE_43','CAN_TX_TRACK_ANGLE_43','CAN_TX_TRACK_STATUS_43','CAN_TX_TRACK_ONCOMING_43','CAN_TX_TRACK_GROUPING_CHANGED_43','CAN_TX_TRACK_LAT_RATE_43'}},'OutputPortsLabelMode','ON','InputPortsWidth',int32(0),'InputPortsActive',0,'DialogFcn','rtican_message_interface_gui','BlockDisplay',{{'','center'}},'IconTransparency','on','ParameterTunableNames',{{}},'InitLevel',3,'BlockName',struct('Token',{{'ESR_Track43'}}),'SampleTime',{{0.01}},'TriggerPort',{{'none'}},'EnablePort',{{'none'}})  RTIBlockParameters=struct('BoardTypeNo',{{1,'OFF',[]}},'BoardNo',{{2,'ON',[1 16]}},'ChannelNo',{{2,'ON',[1 2]}},'Parameters',{{struct('DataFileSupport',struct('DataFileSelectedMaster',1,'DataFileSelectedLocal',0,'DataFileName','c:\users\mpc_car\documents\github\mpc-car\controller\dbcfiles\esr_dv3_64tgt.dbc|','DataFileDate',{{{['02-Nov-2012 20:32:52']},{['21-Mar-2013 13:39:53']},{['28-Sep-2011 17:08:52']}}},'SelectedFile',['<no file selected>'],'InterfaceFcn','rtican_dbc_file_parser'),'Options',struct('StatusSelected',0,'TimeSelected',0,'DeltaTimeSelected',0,'BytePortSelected',0,'MessageLengthSelected',0,'TriggerPort',struct('Selected',0,'TriggerType',0),'UserCoding',struct('Selected',0,'InterfaceFile','UserDecodingFile','FcnName','UserDecodeFcn','InportSelected',0,'InportWidth',1,'OutportSelected',0,'OutportWidth',1),'EnablePortSelected',0,'SignalOnPortnameSelected',1,'UseRXService',0),'Message',struct('MsgOnBlocknameSelected',1,'MsgName','ESR_Track43','MsgIdFormat',0,'MsgId',1322,'MsgLength',8,'NumSignals',12,'SampleTime',0.01,'Signal',struct('SgnName',{'CAN_TX_TRACK_RANGE_RATE_43','CAN_TX_TRACK_MED_RANGE_MODE_43','CAN_TX_TRACK_RANGE_ACCEL_43','CAN_TX_TRACK_WIDTH_43','CAN_TX_TRACK_ROLLING_COUNT_43','CAN_TX_TRACK_BRIDGE_OBJECT_43','CAN_TX_TRACK_RANGE_43','CAN_TX_TRACK_ANGLE_43','CAN_TX_TRACK_STATUS_43','CAN_TX_TRACK_ONCOMING_43','CAN_TX_TRACK_GROUPING_CHANGED_43','CAN_TX_TRACK_LAT_RATE_43'},'SgnStartBit',{0,14,16,26,30,31,32,43,53,56,57,58},'SgnLength',{14,2,10,4,1,1,11,10,3,1,1,6},'SgnType',{0,0,0,0,0,0,0,0,0,0,0,0},'ModeValue',{-1,-1,-1,-1,-1,-1,-1,-1,-1,-1,-1,-1},'DataType',{1,0,1,0,0,0,0,1,0,0,0,1},'ByteLayout',{2,2,2,2,2,2,2,2,2,2,2,2},'Factor',{0.01,1,0.05,0.5,1,1,0.1,0.1,1,1,1,0.25},'Offset',{0,0,0,0,0,0,0,0,0,0,0,0},'SgnComment',{{''},{''},{''},{''},{''},{''},{''},{''},{''},{''},{''},{''}},'SgnUnit',{'m/s','','m/s/s','m','','','m','deg','','','',''},'Min',{-81.92,0,-25.6,0,0,0,0,-51.2,0,0,0,-8},'Max',{81.91,3,25.55,7.5,1,0,204.7,51.1,7,0,0,7.75},'SLDataType',{'SS_DOUBLE','SS_DOUBLE','SS_DOUBLE','SS_DOUBLE','SS_DOUBLE','SS_DOUBLE','SS_DOUBLE','SS_DOUBLE','SS_DOUBLE','SS_DOUBLE','SS_DOUBLE','SS_DOUBLE'}),'MsgIdNumFormat',0,'MsgComment',{{''}}),'Version',1.2,'general',struct('isFromLib',0)),'OFF',[]}},'GroupId',{{struct('Group',{{'RTICAN'}},'No',4,'Behavior',{{'NAMECHANGE'}},'BlockType',{{'SINK'}},'NameChangeFlag',0),'OFF',[]}},'SFcnRTICANMessage',{{struct('MsgType','RX','SFcnPortType','Scalar','MsgName','ESR_Track43','MsgIdFormat','STD','MsgId',1322,'MsgLength',8,'NumSignals',12,'SampleTime',0.01,'Signal',struct('SgnName',{'CAN_TX_TRACK_RANGE_RATE_43','CAN_TX_TRACK_MED_RANGE_MODE_43','CAN_TX_TRACK_RANGE_ACCEL_43','CAN_TX_TRACK_WIDTH_43','CAN_TX_TRACK_ROLLING_COUNT_43','CAN_TX_TRACK_BRIDGE_OBJECT_43','CAN_TX_TRACK_RANGE_43','CAN_TX_TRACK_ANGLE_43','CAN_TX_TRACK_STATUS_43','CAN_TX_TRACK_ONCOMING_43','CAN_TX_TRACK_GROUPING_CHANGED_43','CAN_TX_TRACK_LAT_RATE_43'},'SgnStartBit',{0,14,16,26,30,31,32,43,53,56,57,58},'SgnLength',{14,2,10,4,1,1,11,10,3,1,1,6},'SgnType',{'standard','standard','standard','standard','standard','standard','standard','standard','standard','standard','standard','standard'},'ModeValue',{-1,-1,-1,-1,-1,-1,-1,-1,-1,-1,-1,-1},'DataType',{['signed int'],['unsigned int'],['signed int'],['unsigned int'],['unsigned int'],['unsigned int'],['unsigned int'],['signed int'],['unsigned int'],['unsigned int'],['unsigned int'],['signed int']},'ByteLayout',{['motorola back.'],['motorola back.'],['motorola back.'],['motorola back.'],['motorola back.'],['motorola back.'],['motorola back.'],['motorola back.'],['motorola back.'],['motorola back.'],['motorola back.'],['motorola back.']},'Factor',{0.01,1,0.05,0.5,1,1,0.1,0.1,1,1,1,0.25},'Offset',{0,0,0,0,0,0,0,0,0,0,0,0},'SLDataType',{'SS_DOUBLE','SS_DOUBLE','SS_DOUBLE','SS_DOUBLE','SS_DOUBLE','SS_DOUBLE','SS_DOUBLE','SS_DOUBLE','SS_DOUBLE','SS_DOUBLE','SS_DOUBLE','SS_DOUBLE'}),'StatusSelected','no','TimeSelected','no','DeltaTimeSelected','no','BytePortSelected','no','MessageLengthSelected','no','TriggerPort',struct('Selected','no','TriggerType',0),'UserCoding',struct('Selected','no','InterfaceFile','UserDecodingFile','FcnName','UserDecodeFcn','InportSelected','no','InportWidth',1,'OutportSelected','no','OutportWidth',1),'EnablePortSelected','no','UseRXService','no','BoardType','DS1','BoardNo',2,'ControllerNo',2),'OFF',[]}},'TLCFileName',{{'rtican_rx_message','OFF',[]}})  RTISFcnParameters=struct('SFcnRTICANMessage','struct','TLCFileName','char')  RTIBlockParaDefault=struct('BoardTypeNo',4302,'BoardNo',1,'ChannelNo',1,'Parameters',struct('DataFileSupport',struct('DataFileSelectedMaster',0,'DataFileSelectedLocal',0,'DataFileName','','DataFileDate','','SelectedFile',['<no file selected>']),'Options',struct('StatusSelected',1,'TimeSelected',1,'DeltaTimeSelected',1,'BytePortSelected',0,'MessageLengthSelected',0,'TriggerPort',struct('Selected',0,'TriggerType','rising'),'UserCoding',struct('Selected',0,'InterfaceFile','UserDecodingFile','FcnName','UserDecodeFcn','InportSelected',0,'InportWidth',1,'OutportSelected',0,'OutportWidth',1),'EnablePortSelected',0,'SignalOnPortnameSelected',1,'UseRXService',0),'Message',struct('MsgOnBlocknameSelected',0,'MsgName',['RX Message'],'MsgIdFormat',0,'MsgId',100,'MsgLength',8,'NumSignals',1,'SampleTime',-1,'Signal',struct('SgnName',['RX signal'],'SgnStartBit',0,'SgnLength',8,'SgnType',0,'ModeValue',-1,'DataType',0,'SLDataType','SS_DOUBLE','ByteLayout',0,'Factor',1,'Offset',0,'Min',0,'Max',255,'SgnComment',{{}},'SgnUnit',''),'MsgIdNumFormat',0,'MsgComment',{{''}}),'Version',1.2,'general',struct('isFromLib',1)),'GroupId',struct('Group',{{'RTICAN'}},'No',1,'Behavior',{{'NAMECHANGE'}},'BlockType',{{'SINK'}},'NameChangeFlag',0),'SFcnRTICANMessage',struct('MsgType','RX','MsgName',['RX Message'],'MsgIdFormat','STD','MsgId',100,'MsgLength',8,'NumSignals',1,'SampleTime',-1,'Signal',struct('SgnName',['RX signal'],'SgnStartBit',0,'SgnLength',8,'SgnType','standard','ModeValue',-1,'DataType',['unsigned int'],'ByteLayout',['little endian'],'SLDataType','SS_DOUBLE','Factor',1,'Offset',0),'StatusSelected','yes','TimeSelected','yes','DeltaTimeSelected','yes','BytePortSelected','no','MessageLengthSelected','no','EnablePortSelected','no','UserCoding',struct('Selected','no','InterfaceFile','UserDecodingFile','FcnName','UserDecodeFcn','InportSelected','no','InportWidth',1,'OutportSelected','no','OutportWidth',1),'TriggerPort',struct('Selected','no','TriggerType','rising'),'UseRXService','no','BoardType','DS4302','BoardNo',1,'ControllerNo',1,'SFcnPortType','Scalar'),'TLCFileName','rtican_rx_message')
      settings: AttributesFormatString=Group Id: RTICAN4\n
  Out1 : Outport
  wires:
  Bus Creator/1 -> Out1/1  "Track43"
  ESR_Track43/1 -> Bus Creator/1  "CAN_TX_TRACK_RANGE_RATE_43"
  ESR_Track43/2 -> Bus Creator/2  "CAN_TX_TRACK_MED_RANGE_MODE_43"
  ESR_Track43/3 -> Bus Creator/3  "CAN_TX_TRACK_RANGE_ACCEL_43"
  ESR_Track43/4 -> Bus Creator/4  "CAN_TX_TRACK_WIDTH_43"
  ESR_Track43/5 -> Bus Creator/5  "CAN_TX_TRACK_ROLLING_COUNT_43"
  ESR_Track43/6 -> Bus Creator/6  "CAN_TX_TRACK_BRIDGE_OBJECT_43"
  ESR_Track43/7 -> Bus Creator/7  "CAN_TX_TRACK_RANGE_43"
  ESR_Track43/8 -> Bus Creator/8  "CAN_TX_TRACK_ANGLE_43"
  ESR_Track43/9 -> Bus Creator/9  "CAN_TX_TRACK_STATUS_43"
  ESR_Track43/10 -> Bus Creator/10  "CAN_TX_TRACK_ONCOMING_43"
  ESR_Track43/11 -> Bus Creator/11  "CAN_TX_TRACK_GROUPING_CHANGED_43"
  ESR_Track43/12 -> Bus Creator/12  "CAN_TX_TRACK_LAT_RATE_43"
